simulink subsystem "CustomManeuver"  (R2020a)
settings: Solver=VariableStepAuto  StartTime=0.0  StopTime=10.0  RelTol=1e-3
undefined symbols (not defined in the file or in its folder): SteerRef, xdot_r
libraries: simulink x8
settings Model: Creator=Fil  LastModifiedBy=filip

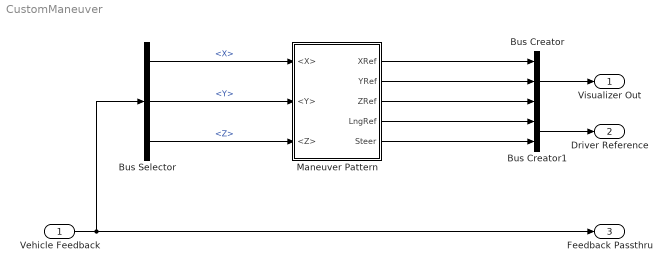
== system CustomManeuver ==
  Vehicle Feedback : Inport
  Bus Creator : BusCreator  Inputs=3
  Bus Creator1 : BusCreator  Inputs=2
  Bus Selector : BusSelector  OutputSignals=Body.X,Body.Y,Body.Z
  Maneuver Pattern : Subsystem  Variant=on  VariantControl=Choice
  Visualizer Out : Outport
  Driver Reference : Outport  Port=2
  Feedback Passthru : Outport  Port=3
  wires:
  Vehicle Feedback/1 -> Feedback Passthru/1, Bus Selector/1
  Bus Creator/1 -> Visualizer Out/1
  Bus Creator1/1 -> Driver Reference/1
  Bus Selector/1 -> Maneuver Pattern/1(<X>)  "<X>"
  Bus Selector/2 -> Maneuver Pattern/2(<Y>)  "<Y>"
  Bus Selector/3 -> Maneuver Pattern/3(<Z>)  "<Z>"
  Maneuver Pattern/1(XRef) -> Bus Creator/1
  Maneuver Pattern/2(YRef) -> Bus Creator/2
  Maneuver Pattern/3(ZRef) -> Bus Creator/3
  Maneuver Pattern/4(LngRef) -> Bus Creator1/1
  Maneuver Pattern/5(Steer) -> Bus Creator1/2

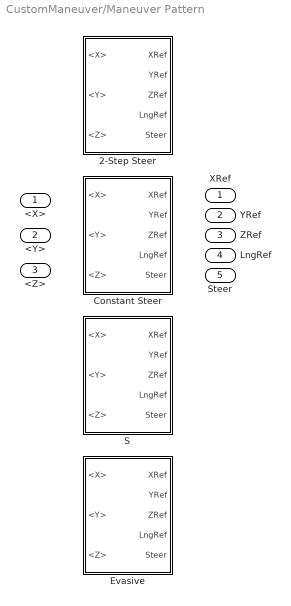
== system CustomManeuver/Maneuver Pattern ==
  <X> : Inport
  <Y> : Inport  Port=2
  <Z> : Inport  Port=3
  2-Step Steer : Subsystem  VariantControl=RefMode == 1
  Constant Steer : Subsystem  VariantControl=RefMode == 0
  Evasive : Subsystem  VariantControl=RefMode == 3
  S : Subsystem  VariantControl=RefMode == 2
  XRef : Outport
  YRef : Outport  Port=2
  ZRef : Outport  Port=3
  LngRef : Outport  Port=4
  Steer : Outport  Port=5

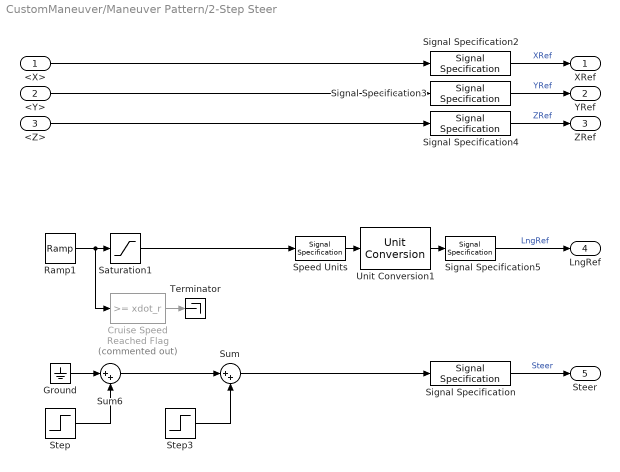
== system CustomManeuver/Maneuver Pattern/2-Step Steer ==
  <X> : Inport
  <Y> : Inport  Port=2
  <Z> : Inport  Port=3
  Cruise Speed Reached Flag : simulink/Logic and Bit Operations/Compare To Constant  Commented=on  relop=>=  const=xdot_r  OutDataTypeStr=boolean
  Ground : Ground
  Ramp1 : simulink/Sources/Ramp  slope=5  start=t_start  InitialOutput=0
  Saturation1 : Saturate  UpperLimit=xdot_r  LowerLimit=0  ZeroCross=off
  Signal Specification : SignalSpecification  Unit=deg
  Signal Specification2 : SignalSpecification
  Signal Specification3 : SignalSpecification
  Signal Specification4 : SignalSpecification
  Signal Specification5 : SignalSpecification  Unit=m/s
  Speed Units : SignalSpecification  Unit=km/h
  Step : Step  Time=20  After=SteerRef  SampleTime=0
  Step3 : Step  Time=23  After=2*SteerRef  SampleTime=0
  Sum : Sum  Inputs=|++
  Sum6 : Sum  Inputs=|++
  Terminator : Terminator
  Unit Conversion1 : UnitConversion
  XRef : Outport
  YRef : Outport  Port=2
  ZRef : Outport  Port=3
  LngRef : Outport  Port=4
  Steer : Outport  Port=5
  wires:
  Sum6/1 -> Sum/1
  Ground/1 -> Sum6/1
  Step/1 -> Sum6/2
  Sum/1 -> Signal Specification/1
  Step3/1 -> Sum/2
  Cruise Speed Reached Flag/1 -> Terminator/1
  Signal Specification2/1 -> XRef/1  "XRef"
  Signal Specification4/1 -> ZRef/1  "ZRef"
  Signal Specification3/1 -> YRef/1  "YRef"
  <Y>/1 -> Signal Specification3/1
  Speed Units/1 -> Unit Conversion1/1
  Unit Conversion1/1 -> Signal Specification5/1
  <X>/1 -> Signal Specification2/1
  Saturation1/1 -> Speed Units/1
  Signal Specification/1 -> Steer/1  "Steer"
  Ramp1/1 -> Saturation1/1, Cruise Speed Reached Flag/1
  <Z>/1 -> Signal Specification4/1
  Signal Specification5/1 -> LngRef/1  "LngRef"

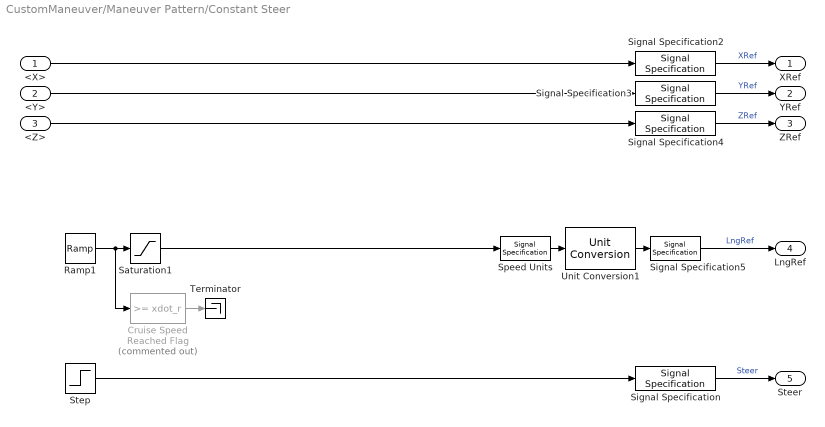
== system CustomManeuver/Maneuver Pattern/Constant Steer ==
  <X> : Inport
  <Y> : Inport  Port=2
  <Z> : Inport  Port=3
  Cruise Speed Reached Flag : simulink/Logic and Bit Operations/Compare To Constant  Commented=on  relop=>=  const=xdot_r  OutDataTypeStr=boolean
  Ramp1 : simulink/Sources/Ramp  slope=5  start=t_start  InitialOutput=0
  Saturation1 : Saturate  UpperLimit=xdot_r  LowerLimit=0  ZeroCross=off
  Signal Specification : SignalSpecification  Unit=deg
  Signal Specification2 : SignalSpecification
  Signal Specification3 : SignalSpecification
  Signal Specification4 : SignalSpecification
  Signal Specification5 : SignalSpecification  Unit=m/s
  Speed Units : SignalSpecification  Unit=km/h
  Step : Step  Time=20  After=SteerRef  SampleTime=0
  Terminator : Terminator
  Unit Conversion1 : UnitConversion
  XRef : Outport
  YRef : Outport  Port=2
  ZRef : Outport  Port=3
  LngRef : Outport  Port=4
  Steer : Outport  Port=5
  wires:
  Cruise Speed Reached Flag/1 -> Terminator/1
  Signal Specification2/1 -> XRef/1  "XRef"
  Signal Specification4/1 -> ZRef/1  "ZRef"
  Signal Specification3/1 -> YRef/1  "YRef"
  <Y>/1 -> Signal Specification3/1
  Speed Units/1 -> Unit Conversion1/1
  Unit Conversion1/1 -> Signal Specification5/1
  <X>/1 -> Signal Specification2/1
  Saturation1/1 -> Speed Units/1
  Step/1 -> Signal Specification/1
  Signal Specification/1 -> Steer/1  "Steer"
  Ramp1/1 -> Saturation1/1, Cruise Speed Reached Flag/1
  <Z>/1 -> Signal Specification4/1
  Signal Specification5/1 -> LngRef/1  "LngRef"

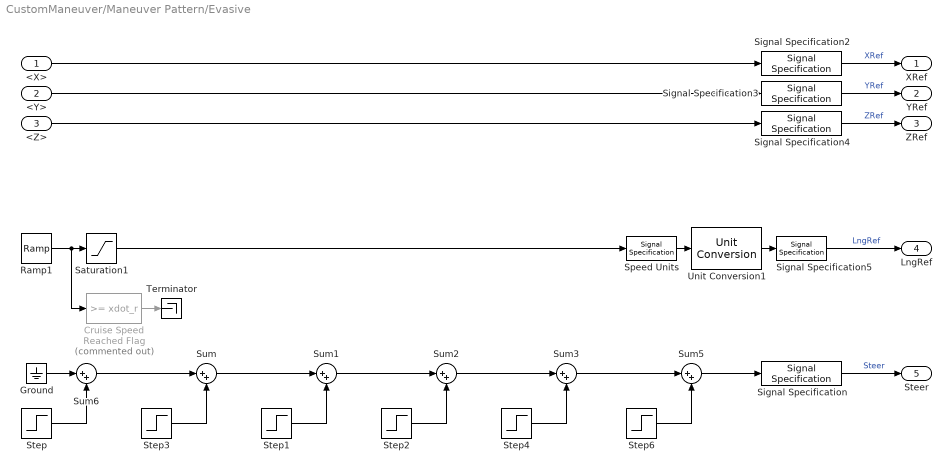
== system CustomManeuver/Maneuver Pattern/Evasive ==
  <X> : Inport
  <Y> : Inport  Port=2
  <Z> : Inport  Port=3
  Cruise Speed Reached Flag : simulink/Logic and Bit Operations/Compare To Constant  Commented=on  relop=>=  const=xdot_r  OutDataTypeStr=boolean
  Ground : Ground
  Ramp1 : simulink/Sources/Ramp  slope=5  start=t_start  InitialOutput=0
  Saturation1 : Saturate  UpperLimit=xdot_r  LowerLimit=0  ZeroCross=off
  Signal Specification : SignalSpecification  Unit=deg
  Signal Specification2 : SignalSpecification
  Signal Specification3 : SignalSpecification
  Signal Specification4 : SignalSpecification
  Signal Specification5 : SignalSpecification  Unit=m/s
  Speed Units : SignalSpecification  Unit=km/h
  Step : Step  Time=20  After=SteerRef  SampleTime=0
  Step1 : Step  Time=22  After=SteerRef  SampleTime=0
  Step2 : Step  Time=24  After=-SteerRef  SampleTime=0
  Step3 : Step  Time=21  After=-2*SteerRef  SampleTime=0
  Step4 : Step  Time=25  After=2*SteerRef  SampleTime=0
  Step6 : Step  Time=26  After=-SteerRef  SampleTime=0
  Sum{,1..3,5..6} (6 alike) : Sum  Inputs=|++
  Terminator : Terminator
  Unit Conversion1 : UnitConversion
  XRef : Outport
  YRef : Outport  Port=2
  ZRef : Outport  Port=3
  LngRef : Outport  Port=4
  Steer : Outport  Port=5
  wires:
  Sum6/1 -> Sum/1
  Ground/1 -> Sum6/1
  Step/1 -> Sum6/2
  Sum5/1 -> Signal Specification/1
  Sum3/1 -> Sum5/1
  Step6/1 -> Sum5/2
  Sum2/1 -> Sum3/1
  Step4/1 -> Sum3/2
  Sum1/1 -> Sum2/1
  Step2/1 -> Sum2/2
  Sum/1 -> Sum1/1
  Step1/1 -> Sum1/2
  Step3/1 -> Sum/2
  Cruise Speed Reached Flag/1 -> Terminator/1
  Signal Specification2/1 -> XRef/1  "XRef"
  Signal Specification4/1 -> ZRef/1  "ZRef"
  Signal Specification3/1 -> YRef/1  "YRef"
  <Y>/1 -> Signal Specification3/1
  Speed Units/1 -> Unit Conversion1/1
  Unit Conversion1/1 -> Signal Specification5/1
  <X>/1 -> Signal Specification2/1
  Saturation1/1 -> Speed Units/1
  Signal Specification/1 -> Steer/1  "Steer"
  Ramp1/1 -> Saturation1/1, Cruise Speed Reached Flag/1
  <Z>/1 -> Signal Specification4/1
  Signal Specification5/1 -> LngRef/1  "LngRef"

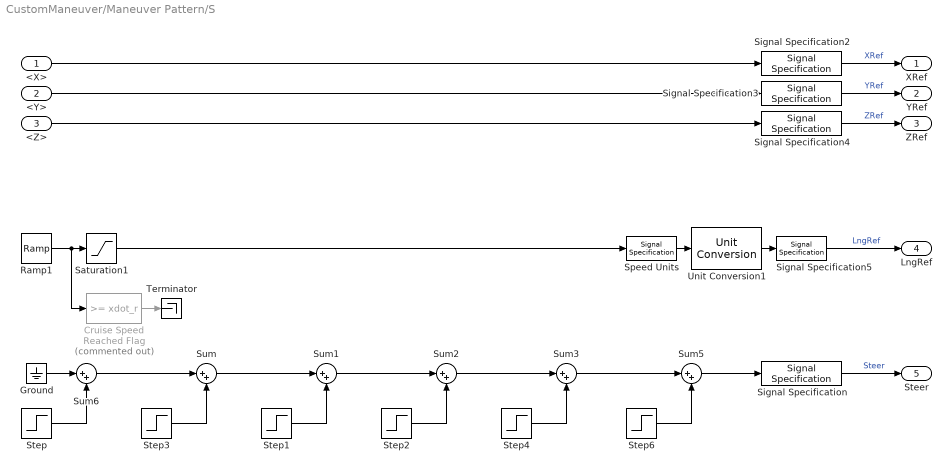
== system CustomManeuver/Maneuver Pattern/S ==
  <X> : Inport
  <Y> : Inport  Port=2
  <Z> : Inport  Port=3
  Cruise Speed Reached Flag : simulink/Logic and Bit Operations/Compare To Constant  Commented=on  relop=>=  const=xdot_r  OutDataTypeStr=boolean
  Ground : Ground
  Ramp1 : simulink/Sources/Ramp  slope=5  start=t_start  InitialOutput=0
  Saturation1 : Saturate  UpperLimit=xdot_r  LowerLimit=0  ZeroCross=off
  Signal Specification : SignalSpecification  Unit=deg
  Signal Specification2 : SignalSpecification
  Signal Specification3 : SignalSpecification
  Signal Specification4 : SignalSpecification
  Signal Specification5 : SignalSpecification  Unit=m/s
  Speed Units : SignalSpecification  Unit=km/h
  Step : Step  Time=20  After=SteerRef  SampleTime=0
  Step1 : Step  Time=24  After=SteerRef  SampleTime=0
  Step2 : Step  Time=34  After=-SteerRef  SampleTime=0
  Step3 : Step  Time=22  After=-2*SteerRef  SampleTime=0
  Step4 : Step  Time=36  After=2*SteerRef  SampleTime=0
  Step6 : Step  Time=38  After=-SteerRef  SampleTime=0
  Sum{,1..3,5..6} (6 alike) : Sum  Inputs=|++
  Terminator : Terminator
  Unit Conversion1 : UnitConversion
  XRef : Outport
  YRef : Outport  Port=2
  ZRef : Outport  Port=3
  LngRef : Outport  Port=4
  Steer : Outport  Port=5
  wires:
  Sum6/1 -> Sum/1
  Ground/1 -> Sum6/1
  Step/1 -> Sum6/2
  Sum5/1 -> Signal Specification/1
  Sum3/1 -> Sum5/1
  Step6/1 -> Sum5/2
  Sum2/1 -> Sum3/1
  Step4/1 -> Sum3/2
  Sum1/1 -> Sum2/1
  Step2/1 -> Sum2/2
  Sum/1 -> Sum1/1
  Step1/1 -> Sum1/2
  Step3/1 -> Sum/2
  Cruise Speed Reached Flag/1 -> Terminator/1
  Signal Specification2/1 -> XRef/1  "XRef"
  Signal Specification4/1 -> ZRef/1  "ZRef"
  Signal Specification3/1 -> YRef/1  "YRef"
  <Y>/1 -> Signal Specification3/1
  Speed Units/1 -> Unit Conversion1/1
  Unit Conversion1/1 -> Signal Specification5/1
  <X>/1 -> Signal Specification2/1
  Saturation1/1 -> Speed Units/1
  Signal Specification/1 -> Steer/1  "Steer"
  Ramp1/1 -> Saturation1/1, Cruise Speed Reached Flag/1
  <Z>/1 -> Signal Specification4/1
  Signal Specification5/1 -> LngRef/1  "LngRef"
